simulink model "RadarSimulinkProjectRev007"  (R2024a)
settings: Solver=VariableStepAuto  StartTime=0.0  StopTime=0.00116  RelTol=1e-3
values from neighbouring files (symbols this model uses):
  AngleTime = SweepTime/10    (= 10000)    [InitializationOfVariables.m]    (also in InitializationOfVariablesRev000.m; InitializationOfVariablesRev001.m; InitializationOfVariablesRev003.m = 2097152; InitializationOfVariablesRev004.m = 2097152)
  ASR_LUT = Rsamp-OffsetDelayR    [InitializationOfVariablesRev003.m]    (also in InitializationOfVariablesRev004.m = round((R*2*SystemFs)/c))
  Btn_Debounce = 20000    [InitializationOfVariablesRev003.m]    (also in InitializationOfVariablesRev004.m)
  ChirpNc = 128    [InitializationOfVariablesRev003.m]    (also in InitializationOfVariablesRev004.m)
  ChirpSizeLength = FreqDeltaPeriod*361    (= 16245)    [InitializationOfVariablesRev003.m]    (also in InitializationOfVariablesRev004.m = 16384)
  DeciFactor = 8    [InitializationOfVariablesRev004.m]
  FCW = [FCW_p1, FCW_p2]    [InitializationOfVariablesRev003.m]    (also in InitializationOfVariablesRev004.m = f / SystemFs)
  filt1divide = sum(h3_int)    [InitializationOfVariablesRev004.m]
  RXFFTLength = 16384    [InitializationOfVariablesRev003.m]    (also in InitializationOfVariablesRev004.m = 2048)
  SweepTime = 100000    [InitializationOfVariables.m]    (also in InitializationOfVariablesRev000.m; InitializationOfVariablesRev001.m; InitializationOfVariablesRev003.m = 23068672; InitializationOfVariablesRev004.m = 23068672)
undefined symbols (not defined in the file or in its folder): SignalGenerationForAnalysis, Subsystem, xc7a200tfbg676
libraries: hdlBasic x383, hdlDSPIP x16, hdlUtilities x11, vmcUtilities x1
(part 1 of 4)
settings Model: Creator=Cube II  LastModifiedBy=Cube II
settings ModelReferenceCC: UpdateModelReferenceTargets=IfOutOfDate

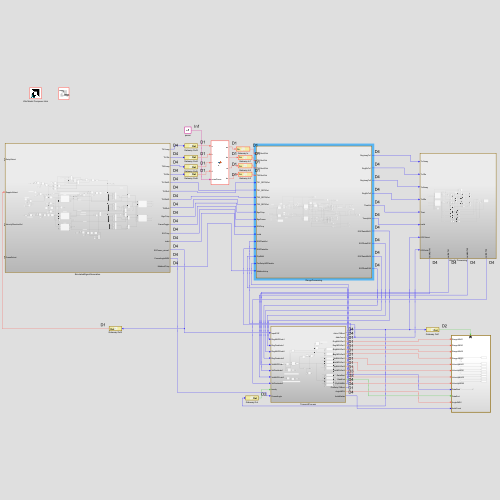
[thumbnail: Simulink's stored preview of the top-level diagram]
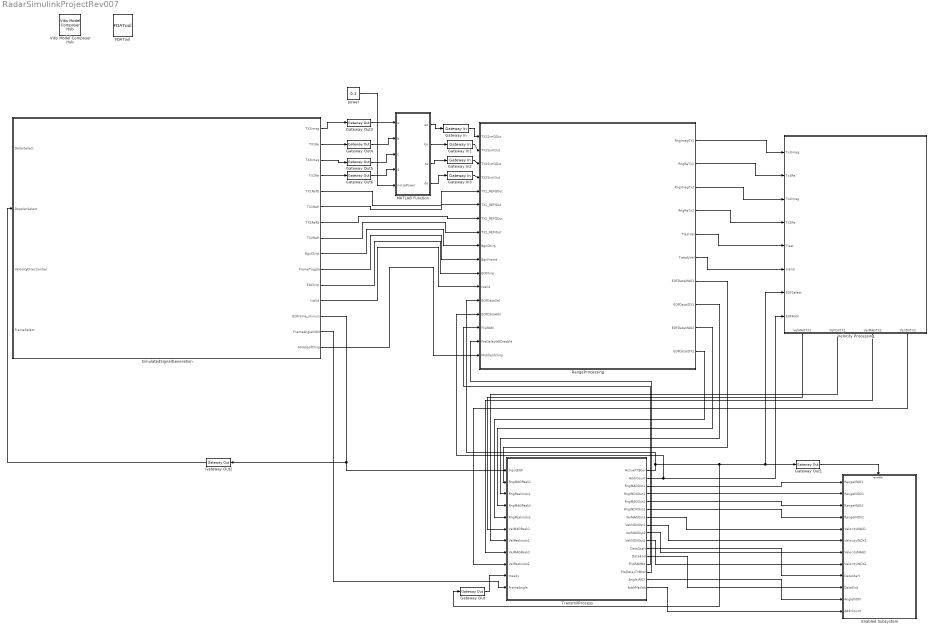
== system RadarSimulinkProjectRev007 ==
  Enabled Subsystem : Subsystem  TreatAsAtomicUnit=on
  FDATool : hdlUtilities/FDATool  block_type=fdatool
      settings: infoedit=FDATool
  Gateway In{,1..3} (4 alike) : hdlBasic/Gateway In  gui_display_data_type=Fixed-point  arith_type=Signed (2's comp)  n_bits=16  bin_pt=14  preci_type=Single  exp_width=8  frac_width=24  rows=1  columns=1  quantization="Round  (unbiased: +/- Inf)"  overflow=Saturate  period=P1  UseAsADC=off  ADCChannel='1'  interface=None  automatic_assignment=on  address_offset=hex2dec('00')  intf_name=''  intf_description=''  default_value=0  timing_constraint=None  locs_specified=off  LOCs={}  io_standard={}  inherit_from_input=off  hdl_port=on  XmcBlockStatus=1  maskContainerNames=group4  block_type=gatewayin  block_config=sysgen:gateway_in_config  block_width_w=590  block_height_w=620  block_width=640  block_height=850
  Gateway Out{,1..6} (7 alike) : hdlBasic/Gateway Out  inherit_from_input=off  bool_to_boolean=off  hdl_port=on  rows=1  columns=1  UseAsDAC=off  DACChannel='1'  interface=None  automatic_assignment=on  address_offset=hex2dec('00')  intf_name=''  intf_description=''  timing_constraint=None  locs_specified=off  LOCs={}  io_standard={}  XmcBlockStatus=1  maskContainerNames=group4  block_type=gatewayout  block_config=sysgen:gateway_out_config  block_width_w=590  block_height_w=620  block_width=620  block_height=750
  MATLAB Function : MATLAB Function  TreatAsAtomicUnit=on
  RangeProcessing : Subsystem
  SimulatedSignalGeneration : Subsystem  SystemSampleTime=1/200e6
  TransmitProcess : Subsystem
  Velocity Processing : Subsystem
      settings: PortSchema="{\"entries\":[{\"content\":{\"sides\":[{\"content\":{\"connectorIds\":[\"In1\",\"In2\",\"In3\",\"In4\",\"In5\",\"In6\",\"In7\",\"In8\"]},\"type\":\"ConnectorPlacement.EquallySpacedRectSide\",\"uuid\":\"28660edc-4300-4d13-b5c7-cb230341ceef\"},{\"content\":{\"side\":\"RIGHT\"},\"type\":\"ConnectorPlacement.EquallySpacedRectSide\",\"uuid\":\"0aea0b64-dbd9-49d9-980c-6712e9fa4544\"},{\"content\":{\"side\":\"TOP\"},\"type\":\"ConnectorPlacement.EquallySpacedRectSide\",\"uuid\":\"4015706e-c6eb-4ca9-b4bb-31c510b09214\"},{\"content\":{\"connectorIds\":[\"Out1\",\"Out2\",\"Out3\",\"Out4\"],\"side\":\"BOTTOM\"},\"type\":\"ConnectorPlacement.EquallySpacedRectSide\",\"uuid\":\"e3ca7ed1-345c-4783-9732-f7a0ff2c5995\"}]},\"type\":\"ConnectorPlacement.EquallySpacedConnector\",\"uuid\":\"ab051aed-e004-4640-a7d2-fe89028938d7\"}],\"packageUris\":[\"http://schema.mathworks.com/mf0/Connector/R2020b\"],\"version\":\"1.0\"}"
  Vitis Model Composer Hub : vmcUtilities/Vitis Model Composer Hub  Tag=genX  CodeGeneration=off  SubsystemName=RangeProcessing  BlockHierPath=SignalGenerationForAnalysis/Subsystem  CompilationType=HDLCompilation  SubsystemType=HDLNode  ExportTypeV2=IP Catalog  StartColumn=1  NumberOfColumns=1  TargetDirectory=./netlist  exportDesign=off  analyzeDesign=on  validateDesignOnHw=off  ExportType=AI Engines  IpVendor=xilinx.com  IpLibrary=hls  IpVersion=1.0  IpHWLanguage=Verilog  AieCompilerOptions={}  AieSimulatorOptions={}  CreateTestbench=on  TestbenchStackSize=10  RunRtlSim=off  RunCSim=off  RunAieSim=off  AieSimTimeout=50000  RunAieSimProfiling=off  LaunchVitisAnalyzer=off  PlotOutput=off  RunX86Sim=off  X86SimTimeout=10  GenHwImage=off  GenLibadfXo=on  GenHwValidationCode=off  PlatformType=Not Specified  HwSystemType=Baremetal  HwValidationTarget=hw  ProjDevice=Artix-7 AC701 Evaluation Platform (xc7a200tfbg676-2)  ProjDevicePart=xc7a200tfbg676-2  AIEType=None  SamplePeriod=-1  ClockFrequency=200  DataPathParallelism=1  xilinxfamily=artix7  part=xc7a200t  speed=-2  package=fbg676  directory=./netlist\ip\RangeProcessing\src  testbench=off  incr_netlist=off  synthesis_tool=Vivado  clock_wrapper=Clock Enables  dbl_ovrd=According to Block Masks  dcm_input_clock_period=10  sysclk_period=6.25  simulink_period=1/192e6  eval_field=0  IPInfoJsonString="{\"DUTSubsystemName\":\"Subsystem\",\"HDLSubsystem\":{\"SubsystemName\":\"Subsystem\",\"IPName\":\"Subsystem\",\"IPLibrary\":\"VMC\",\"IPVendor\":\"User Company\",\"IPVersion\":\"1.0\",\"TargetDirectory\":\"./netlist\",\"SubsystemDir\":\"./netlist\\\\ip\\\\Subsystem\",\"FreqHz\":\"200000000\"},\"SubsystemTag\":\"HDLNode\"}"  LogFileName=S:\RadarProjectSimulink\netlist\model_composer.log  NThreads=4  IPConfigFile=C:\Users\Cube II\AppData\Local\Temp\vmctmp-5941030035629153029\SignalGenerationForAnalysis_ipconfig.json
  power : Constant  Value=0.1
  wires:
  SimulatedSignalGeneration/3(TX2Imag) -> Gateway Out5/1
  SimulatedSignalGeneration/7(TX2RefQ) -> RangeProcessing/7(TX2_REFQOut)
  SimulatedSignalGeneration/8(TX2RefI) -> RangeProcessing/8(TX2_REFIOut)
  SimulatedSignalGeneration/10(FrameToggle) -> RangeProcessing/10(BgnFrame)
  SimulatedSignalGeneration/9(BgnChirp) -> RangeProcessing/9(BgnChirp)
  SimulatedSignalGeneration/2(TX1Re) -> Gateway Out4/1
  SimulatedSignalGeneration/1(TX1Imag) -> Gateway Out3/1
  SimulatedSignalGeneration/6(TX1RefI) -> RangeProcessing/6(TX1_REFIOut)
  SimulatedSignalGeneration/5(TX1RefQ) -> RangeProcessing/5(TX1_REFQOut)
  SimulatedSignalGeneration/11(EOChirp) -> RangeProcessing/11(EOChirp)
  SimulatedSignalGeneration/12(tvalid) -> RangeProcessing/12(tvalid)
  RangeProcessing/1(RngImagTx1) -> Velocity Processing/1(Tx1Imag)
  RangeProcessing/2(RngReTx1) -> Velocity Processing/2(Tx1Re)
  RangeProcessing/3(RngImagTx2) -> Velocity Processing/3(Tx2Imag)
  RangeProcessing/4(RngReTx2) -> Velocity Processing/4(Tx2Re)
  RangeProcessing/5(TlastVel) -> Velocity Processing/5(Tlast)
  RangeProcessing/6(TreadyVel) -> Velocity Processing/6(tvalid)
  SimulatedSignalGeneration/13(EOFrame_minus1) -> TransmitProcess/1(InputEOF), Gateway Out2/1
  TransmitProcess/1(ActiveTXBool) -> RangeProcessing/13(EOFDataSel), Gateway Out/1, Gateway Out1/1, Velocity Processing/7(EOFSelect)
  TransmitProcess/2(AddrCount) -> RangeProcessing/14(EOFDataAdrr), Velocity Processing/8(EOFAddr)
  RangeProcessing/7(EOFDataMAG1) -> TransmitProcess/2(RngMAGPeak1)
  RangeProcessing/8(EOFDataIDX1) -> TransmitProcess/3(RngPeakIndx1)
  RangeProcessing/9(EOFDataMAG2) -> TransmitProcess/4(RngMAGPeak2)
  RangeProcessing/10(EOFDataIDX2) -> TransmitProcess/5(RngPeakindx2)
  Velocity Processing/1(VelMAGTX1) -> TransmitProcess/6(VelMAGPeak1)
  Velocity Processing/2(VelIDXTX1) -> TransmitProcess/7(VelPeakIndx1)
  Velocity Processing/3(VelMAGTX2) -> TransmitProcess/8(VelMAGPeak2)
  Velocity Processing/4(VelIDXTX2) -> TransmitProcess/9(VelPeakindx2)
  Gateway Out/1 -> TransmitProcess/10(tready)
  TransmitProcess/13(FlipRAMBit) -> RangeProcessing/15(FlipRAM)
  TransmitProcess/14(PreDelayTXBool) -> RangeProcessing/16(PreDelayWEDisable)
  TransmitProcess/3(RngMAGOut1) -> Enabled Subsystem/1(RangeMAG1)
  TransmitProcess/4(RngINDXOut1) -> Enabled Subsystem/2(RangeINDX1)
  TransmitProcess/5(RngMAGOut2) -> Enabled Subsystem/3(RangeMAG2)
  TransmitProcess/6(RngINDXOut2) -> Enabled Subsystem/4(RangeINDX2)
  TransmitProcess/7(VelMAGOut1) -> Enabled Subsystem/5(VelocityMAG1)
  TransmitProcess/8(VelINDXOut1) -> Enabled Subsystem/6(VelocityINDX1)
  TransmitProcess/9(VelMAGOut2) -> Enabled Subsystem/7(VelocityMAG2)
  TransmitProcess/10(VelINDXOut2) -> Enabled Subsystem/8(VelocityINDX2)
  TransmitProcess/11(DataStart) -> Enabled Subsystem/9(DataStart)
  TransmitProcess/12(DataEnd) -> Enabled Subsystem/10(DataEnd)
  Gateway Out1/1 -> Enabled Subsystem/Enable
  SimulatedSignalGeneration/14(FrameAngleINDX) -> TransmitProcess/11(FrameAngle)
  TransmitProcess/15(AngleINDX) -> Enabled Subsystem/11(AngleINDX)
  TransmitProcess/16(AddrMatlab) -> Enabled Subsystem/12(AddrCount)
  Gateway Out2/1 -> SimulatedSignalGeneration/2(DopplerSelect)
  MATLAB Function/1(ao) -> Gateway In/1
  Gateway Out3/1 -> MATLAB Function/1(a)
  Gateway In/1 -> RangeProcessing/1(TX1SimQOut)
  power/1 -> MATLAB Function/5(noisePower)
  Gateway In1/1 -> RangeProcessing/2(TX1SimIOut)
  Gateway Out4/1 -> MATLAB Function/2(b)
  MATLAB Function/2(bo) -> Gateway In1/1
  Gateway In2/1 -> RangeProcessing/3(TX2SimQOut)
  Gateway In3/1 -> RangeProcessing/4(TX2SimIOut)
  SimulatedSignalGeneration/4(TX2Re) -> Gateway Out6/1
  Gateway Out5/1 -> MATLAB Function/3(c)
  Gateway Out6/1 -> MATLAB Function/4(d)
  MATLAB Function/3(co) -> Gateway In2/1
  MATLAB Function/4(do) -> Gateway In3/1
  SimulatedSignalGeneration/15(MiddleofChirp) -> RangeProcessing/17(Middleofchirp)

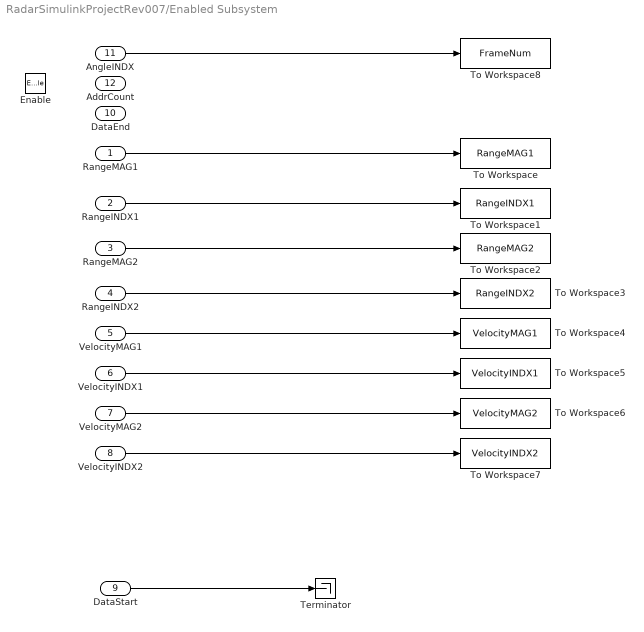
== system RadarSimulinkProjectRev007/Enabled Subsystem ==
  RangeMAG1 : Inport
  RangeINDX1 : Inport  Port=2
  RangeMAG2 : Inport  Port=3
  RangeINDX2 : Inport  Port=4
  VelocityMAG1 : Inport  Port=5
  VelocityINDX1 : Inport  Port=6
  VelocityMAG2 : Inport  Port=7
  VelocityINDX2 : Inport  Port=8
  DataStart : Inport  Port=9
  DataEnd : Inport  Port=10
  AngleINDX : Inport  Port=11
  AddrCount : Inport  Port=12
  Enable : EnablePort
  Terminator : Terminator
  To Workspace : ToWorkspace  VariableName=RangeMAG1  SampleTime=-1
      settings: Save2DSignal=2-D array (concatenate along first dimension)
  To Workspace1 : ToWorkspace  VariableName=RangeINDX1  SampleTime=-1
      settings: Save2DSignal=2-D array (concatenate along first dimension)
  To Workspace2 : ToWorkspace  VariableName=RangeMAG2  SampleTime=-1
      settings: Save2DSignal=2-D array (concatenate along first dimension)
  To Workspace3 : ToWorkspace  VariableName=RangeINDX2  SampleTime=-1
      settings: Save2DSignal=2-D array (concatenate along first dimension)
  To Workspace4 : ToWorkspace  VariableName=VelocityMAG1  SampleTime=-1
      settings: Save2DSignal=2-D array (concatenate along first dimension)
  To Workspace5 : ToWorkspace  VariableName=VelocityINDX1  SampleTime=-1
      settings: Save2DSignal=2-D array (concatenate along first dimension)
  To Workspace6 : ToWorkspace  VariableName=VelocityMAG2  SampleTime=-1
      settings: Save2DSignal=2-D array (concatenate along first dimension)
  To Workspace7 : ToWorkspace  VariableName=VelocityINDX2  SampleTime=-1
      settings: Save2DSignal=2-D array (concatenate along first dimension)
  To Workspace8 : ToWorkspace  VariableName=FrameNum  SampleTime=-1
      settings: Save2DSignal=2-D array (concatenate along first dimension)
  wires:
  DataStart/1 -> Terminator/1
  RangeMAG2/1 -> To Workspace2/1
  RangeINDX2/1 -> To Workspace3/1
  VelocityMAG1/1 -> To Workspace4/1
  VelocityINDX1/1 -> To Workspace5/1
  VelocityMAG2/1 -> To Workspace6/1
  VelocityINDX2/1 -> To Workspace7/1
  AngleINDX/1 -> To Workspace8/1
  RangeMAG1/1 -> To Workspace/1
  RangeINDX1/1 -> To Workspace1/1
